simulink model "simulink_motor_control"  (R2024b)
settings: Solver=VariableStepAuto  StartTime=0.0  StopTime=20  MaxStep=0.001  RelTol=1e-3
values from neighbouring files (symbols this model uses):
  fc = 40    [SampleCodeCSD_CRP.m]    (also in data for tf of motor 2.mat; data for tf of motor 3.mat; data for tf of motor.mat)
  Ts = 1/fs    (= 0.0125)    [SampleCodeCSD_CRP.m]    (also in data for tf of motor 2.mat; data for tf of motor 3.mat; data for tf of motor.mat)
settings Model: Creator=DONGMO ZEWO  LastModifiedBy=DONGMO ZEWO

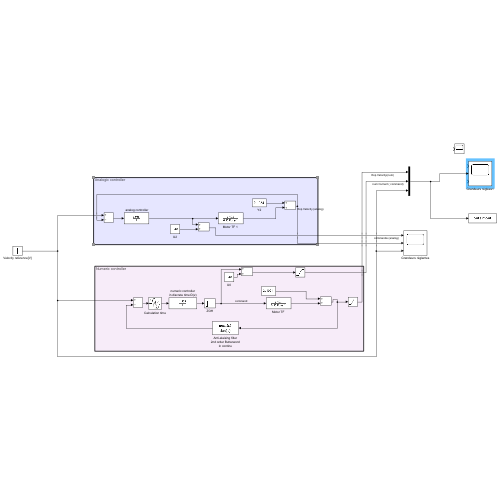
[thumbnail: Simulink's stored preview of the top-level diagram]
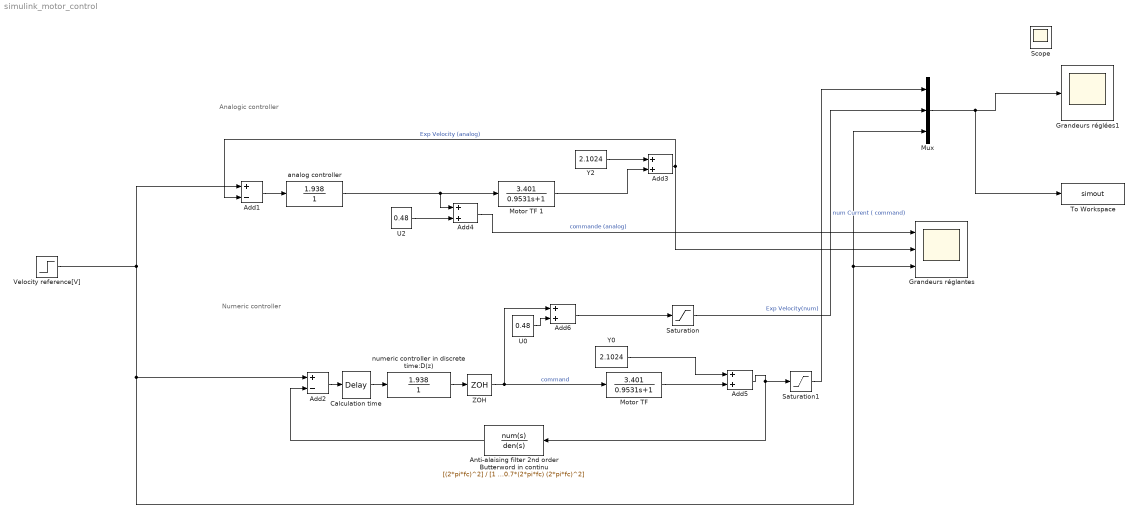
== system simulink_motor_control ==
  note: Analogic controller
  note: Numeric controller
  " analog controller" : TransferFcn  Numerator=[1.938]  Denominator=[1]
  Add1 : Sum  Inputs=+-
  Add2 : Sum  Inputs=+-
  Add{3..6} (4 alike) : Sum
  Anti-alaising filter 2nd order Butterword in continu : TransferFcn  Numerator=[(2*pi*fc)^2]  Denominator=[1 2*0.7*(2*pi*fc) (2*pi*fc)^2]
  Calculation time : TransportDelay  DelayTime=Ts/2
  Grandeurs réglantes : Scope  NumInputPorts=3
  Grandeurs réglées1 : Scope  NumInputPorts=3
  "Motor TF " : TransferFcn  Numerator=[3.401]  Denominator=[0.9531 1]
  "Motor TF 1 " : TransferFcn  Numerator=[3.401]  Denominator=[0.9531 1]
  Mux : Mux  Inputs=3
  Saturation : Saturate  UpperLimit=9  LowerLimit=-9
  Saturation1 : Saturate  UpperLimit=7  LowerLimit=-7
  Scope : Scope
  To Workspace : ToWorkspace  VariableName=simout  SaveFormat=Timeseries  SampleTime=-1
  U0 : Constant  Value=0.48
  U2 : Constant  Value=0.48
  Velocity reference[V] : Step  Time=5  Before=2.1024  After=4  SampleTime=0
  Y0 : Constant  Value=2.1024
  Y2 : Constant  Value=2.1024
  ZOH : ZeroOrderHold  SampleTime=Ts
  numeric controller in discrete time:D(z) : DiscreteTransferFcn  Numerator=1.938  Denominator=[1]  SampleTime=Ts
  wires:
  Add4/1 -> Grandeurs réglantes/1  "commande (analog)"
  " analog controller"/1 -> Add4/1, "Motor TF 1 "/1
  U2/1 -> Add4/2
  Add1/1 -> " analog controller"/1
  Add3/1 -> Add1/2, Grandeurs réglantes/2  "Exp Velocity (analog)"
  Y2/1 -> Add3/1
  Mux/1 -> To Workspace/1, Grandeurs réglées1/2
  "Motor TF 1 "/1 -> Add3/2
  Add2/1 -> Calculation time/1
  Velocity reference[V]/1 -> Add1/1, Add2/1, Grandeurs réglantes/3, Mux/3
  "Motor TF "/1 -> Add5/2
  Add5/1 -> Anti-alaising filter 2nd order Butterword in continu/1, Saturation1/1
  numeric controller in discrete time:D(z)/1 -> ZOH/1
  ZOH/1 -> "Motor TF "/1, Add6/1  "command"
  U0/1 -> Add6/2
  Anti-alaising filter 2nd order Butterword in continu/1 -> Add2/2
  Add6/1 -> Saturation/1
  Y0/1 -> Add5/1
  Calculation time/1 -> numeric controller in discrete time:D(z)/1
  Saturation/1 -> Mux/2  "num Current ( command)"
  Saturation1/1 -> Mux/1  "Exp Velocity(num)"
